simulink model "AUVenv"  (R2026a)
settings: Solver=FixedStepAuto  StopTime=Inf  FixedStep=0.01
PostLoadFcn:
  | set_param(gcs,'Zoomfactor','fit to view')
undefined symbols (not defined in the file or in its folder): AUV, fractalcoef, Sim3dSensor, Simple, T200, thrust_pwms, thruster_pose, XYZ
libraries: sim3dlib x7, robotcorelib x5, AUVLib x4, aerolib6dof2 x2, sim3dcameralib x2, matrix_library x1, mspsensorlib x1, aerolibutil x1
(part 2 of 2)

== matlab function AUVenv/AUVSimu/Sensors/DVL ==
  settings: updateMethod=DISCRETE
  data: body_vel input; vel_b_dvl output; position_e input; rot_m input; v_current_e input; reference_mode input; altitude_dvl output; vel_cov_diag_dvl output; reference output
function [vel_b_dvl, altitude_dvl, vel_cov_diag_dvl, reference] = dvl_sim(body_vel, position_e, rot_m, v_current_e, reference_mode)

seafloor_depth = 2.25; %Depth of pool in m
depth = position_e(3) + 2.2;

vel_b_dvl = zeros([3,1]);

% Noise (1-sigma) in m/s; typical small DVL ~ 0.003–0.02 m/s
sigma_xyz = [0.01; 0.01; 0.015];


% Slow bias as Gauss-Markov (per axis)
tau_bias = 300.0;         % s, time constant of bias drift (5 min)
sigma_bias_ss = 0.01;     % m/s, steady-state std dev of bias
dt = 0.01;                % s, assumed sample time for bias update


persistent bxyz
if isempty(bxyz)
    bxyz = zeros(3,1);
end

v_b_true = body_vel;

reference = uint8(reference_mode);
if reference == uint8(1) % bottom-track
    v_rel_b = v_b_true;
elseif reference == uint8(2) % water-track
    v_rel_b = v_b_true + (rot_m * v_current_e);
else
    % Unknown: default to bottom-track behavior
    v_rel_b = v_b_true;
    reference = uint8(0);
end

if ~isnan(depth) && ~isnan(seafloor_depth)
    altitude_dvl = max(seafloor_depth - depth, 0.0);
else
    altitude_dvl = NaN;
end

% ---------------- Update bias (Gauss-Markov) ----------------
if tau_bias > 0 && sigma_bias_ss > 0
    % Discrete-time OU: b_{k+1} = (1 - dt/tau) b_k + sqrt(2*sigma^2*dt/tau) * w
    a = max(0.0, 1.0 - dt/tau_bias);
    q = sqrt(max(0.0, 2.0*sigma_bias_ss^2*dt/tau_bias));
    bxyz = a*bxyz + q * randn(3,1);
else
    bxyz = zeros(3,1);
end

% ---------------- Add noise & bias ----------------
eps_xyz = sigma_xyz .* randn(3,1);    % white noise
vel_b_dvl = v_rel_b + bxyz + eps_xyz;

vel_cov_diag_dvl = sigma_xyz.^2;

== matlab function AUVenv/AUVSimu/Actuators/Marker/Marker Dynamics/MATLAB Function ==
  data: init_pos input; init_velocity input; marker_position output; rot_m input; marker_loc_b input
function marker_position = marker_traj(init_pos, init_velocity, rot_m, marker_loc_b)

%Get initial position in inertial frame
position_0 = (eye(3)\rot_m)*marker_loc_b + init_pos;

g = 9.79624;
a = [0 0 g]';

persistent position_t
if isempty(position_t)
    position_t = position_0;
end

persistent velocity
if isempty(velocity)
    velocity = init_velocity;
end

%sample time
dt = 0.01;

% Update position using Newton's equations of motion
% position_t(1) = position_t(1) + velocity(1)*dt;
% position_t(2) = position_t(2) + velocity(2)*dt;
% position_t(3) = position_t(3) + velocity(3)*dt + 0.5*g*dt^2;
position_t = position_t + velocity.*dt + 0.5.*a.*dt^2;

% Velocity updated with uniform drag in all axes (assuming a sphere)
velocity = velocity + a.*dt - (diag([0.02 0.02 0.02]) * velocity);

% set z position to pool floor once it reaches/exceeds pool depth
if position_t(3) > 0.4
    position_t(3) = 0.4;
end

marker_position = position_t;
